simulink model "tut3"  (R2022a)
settings: Solver=FixedStepAuto  StartTime=0.0  StopTime=10.0  FixedStep=1e-3  RelTol=1e-3  EnableMultiTasking=on
libraries: frdmk64flib x5, etargetslib x2
settings Model: ExtModeTrigDuration=5  Creator=gurle  LastModifiedBy=gurle
settings OptimizationCC: EnhancedBackFolding=on  PassReuseOutputArgsAs=Individual arguments  ZeroExternalMemoryAtStartup=off  ZeroInternalMemoryAtStartup=off  MaxStackSize=64  OptimizeBlockOrder=speed  DifferentSizesBufferReuse=on  OptimizationCustomize=off  EfficientTunableParamExpr=on
settings DebuggingCC: ParameterTunabilityLossMsg=error
settings HardwareCC: ProdBitPerPointer=32  ProdBitPerSizeT=32  ProdBitPerPtrDiffT=32  ProdLargestAtomicInteger=Long  ProdLargestAtomicFloat=Double  ProdWordSize=32  ProdHWDeviceType=ARM Compatible->ARM Cortex
settings SFSimCC: MATLABDynamicMemAlloc=off
settings RTWCC: SystemTargetFile=ert.tlc  HardwareBoard=NXP FRDM-K64F  TLCOptions="-aInlineSetEventsForThisBaseRateFcn=TLC_FALSE -aSuppressMultiTaskScheduler=TLC_FALSE  -aRateBasedStepFcn=0"  TemplateMakefile=ert_default_tmf  Toolchain=GNU Tools for ARM Embedded Processors
settings CodeAppCC: ForceParamTrailComments=on  IgnoreCustomStorageClasses=off  OperatorAnnotations=on  SimulinkDataObjDesc=on  SFDataObjDesc=on  InsertBlockDesc=on
settings ERTTargetCC: ExtModeTransport=4  ExtModeMexFile=sendToCommService

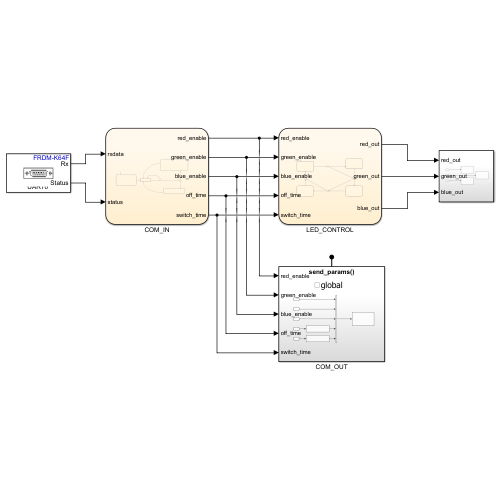
[thumbnail: Simulink's stored preview of the top-level diagram]
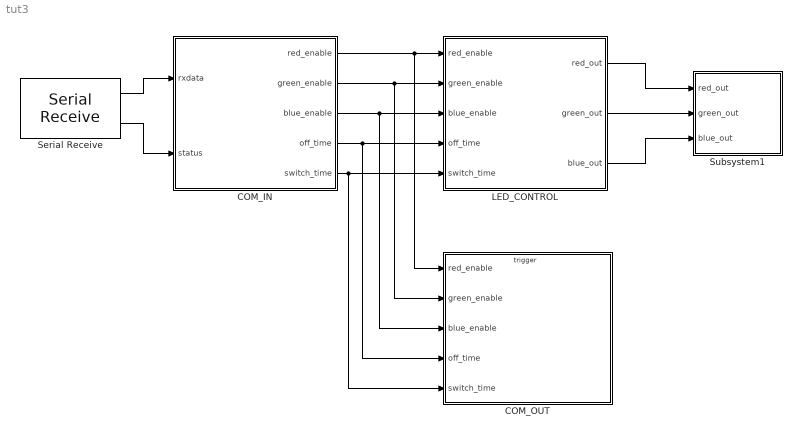
== system tut3 ==
  COM_IN : Stateflow chart  TreatAsAtomicUnit=on
  COM_OUT : Subsystem  TreatAsAtomicUnit=on
  LED_CONTROL : Stateflow chart  TreatAsAtomicUnit=on
  Serial Receive : frdmk64flib/Serial Receive  SCIModule=0  Baudrate=uint32(9600)  Parity=None  StopBits=1  HardwareFlowControl=None  ByteOrder=LittleEndian  DataType=uint8  DataLength=11  BlockingMode=off  OutputStatus=on  SampleTime=-1
  Subsystem1 : Subsystem
  wires:
  Serial Receive/2 -> COM_IN/2(status)
  Serial Receive/1 -> COM_IN/1(rxdata)
  COM_IN/1(red_enable) -> COM_OUT/1(red_enable), LED_CONTROL/1(red_enable)
  COM_IN/2(green_enable) -> COM_OUT/2(green_enable), LED_CONTROL/2(green_enable)
  COM_IN/3(blue_enable) -> COM_OUT/3(blue_enable), LED_CONTROL/3(blue_enable)
  COM_IN/4(off_time) -> COM_OUT/4(off_time), LED_CONTROL/4(off_time)
  COM_IN/5(switch_time) -> COM_OUT/5(switch_time), LED_CONTROL/5(switch_time)
  LED_CONTROL/1(red_out) -> Subsystem1/1(red_out)
  LED_CONTROL/2(green_out) -> Subsystem1/2(green_out)
  LED_CONTROL/3(blue_out) -> Subsystem1/3(blue_out)

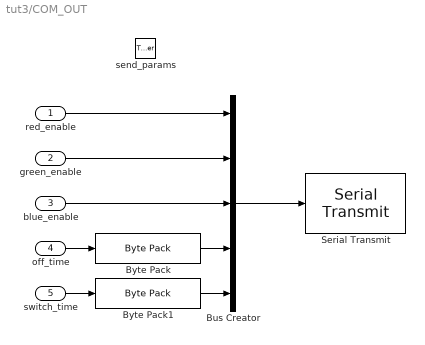
== system tut3/COM_OUT ==
  red_enable : Inport
  green_enable : Inport  Port=2
  blue_enable : Inport  Port=3
  off_time : Inport  Port=4
  switch_time : Inport  Port=5
  send_params : TriggerPort  TriggerType=function-call  IsSimulinkFunction=on  FunctionName=send_params  VariantControl=(inherit)
  Bus Creator : BusCreator  Inputs=5
  Byte Pack : etargetslib/Byte Pack  datatypes={'double'}  byteAlign=1
  Byte Pack1 : etargetslib/Byte Pack  datatypes={'double'}  byteAlign=1
  Serial Transmit : frdmk64flib/Serial Transmit  SCIModule=0  Baudrate=uint32(9600)  Parity=None  StopBits=1  HardwareFlowControl=None  ByteOrder=LittleEndian  BlockingMode=on  OutputStatus=off
  wires:
  Byte Pack1/1 -> Bus Creator/5
  off_time/1 -> Byte Pack/1
  blue_enable/1 -> Bus Creator/3
  Bus Creator/1 -> Serial Transmit/1
  red_enable/1 -> Bus Creator/1
  switch_time/1 -> Byte Pack1/1
  green_enable/1 -> Bus Creator/2
  Byte Pack/1 -> Bus Creator/4

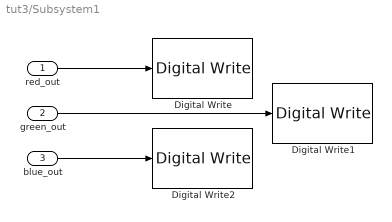
== system tut3/Subsystem1 ==
  red_out : Inport
  green_out : Inport  Port=2
  blue_out : Inport  Port=3
  Digital Write : frdmk64flib/Digital Write  Whichpin=RED_LED
  Digital Write1 : frdmk64flib/Digital Write  Whichpin=GREEN_LED
  Digital Write2 : frdmk64flib/Digital Write  Whichpin=BLUE_LED
  wires:
  green_out/1 -> Digital Write1/1
  red_out/1 -> Digital Write/1
  blue_out/1 -> Digital Write2/1

== stateflow chart tut3/COM_IN ==
  settings: executeAtInitialization=1
  state SET_PARAM
    entry:
    red_enable = rxdata(3);
    green_enable = rxdata(4);
    blue_enable = rxdata(5);
    off_time = typecast(rxdata(6:9), 'single');
    switch_time = typecast(rxdata(10:11), 'unit16');
  state INITIAL
    entry:
    red_enable = 1;
    green_enable = 1;
    blue_enable = 0;
    off_time = 0.5;
    switch_time = 200;
  state STANDBY
  state ECHO_PARAM
    entry:
    send_params();
  SET_PARAM -> STANDBY
  (junction 23) -> SET_PARAM [order 1] : [rxdata(2) = hex2dec('55')]
  (default) -> INITIAL
  (junction 20) -> STANDBY [order 1]
  INITIAL -> STANDBY
  STANDBY -> (junction 20) : [status == 0]
  (junction 20) -> (junction 23) [order 2] : [rxdata(1) == hex2dec('16)]
  (junction 23) -> ECHO_PARAM [order 2] : [rxdata)2_ == hex2dec('22')]
  ECHO_PARAM -> STANDBY
  data: rxdata input; status input; red_enable output; green_enable output; blue_enable output; off_time output; switch_time output

== stateflow chart tut3/LED_CONTROL ==
  state RED_ON
    entry:
    red_out = 1;
    green_out = 0;
    blue_out = 0;
  state OFF
    entry:
    red_out = 0;
    green_out = 0;
    blue_out = 0;
  state BLUE_ON
    entry:
    red_out = 0;
    green_out = 0;
    blue_out = 1;
  state GREEN_ON
    entry:
    red_out = 0;
    green_out = 1;
    blue_out = 0;
  (default) -> OFF
  OFF -> (junction 26) : after(off_time_sec)
  (junction 26) -> RED_ON [order 1] : [red_enable == 1]
  (junction 26) -> (junction 23) [order 2]
  RED_ON -> (junction 23) : after(off_time_sec)
  (junction 17) -> OFF
  (junction 23) -> (junction 20) [order 2]
  (junction 20) -> (junction 17) [order 2]
  BLUE_ON -> (junction 17) : after(off_time_sec)
  (junction 23) -> GREEN_ON [order 1] : [green_enable == 1]
  (junction 20) -> BLUE_ON [order 1] : [blue_enable == 1]
  GREEN_ON -> (junction 20) : after(off_time_sec)
  data: red_enable input; green_enable input; blue_enable input; off_time input; switch_time input; red_out output; green_out output; blue_out output
